simulink model "Part2_Solution"  (R2025a)
settings: Solver=VariableStepAuto  StopTime=5000
InitFcn:
  | addpath(fullfile(fileparts(get_param(bdroot,'FileName')),'..','..','AIEngine_Library','common','matlab')); CreateFilter;
undefined symbols (not defined in the file): Asymmetric, cfi, hb1, hb2, hb3, S, Shift1, Shift2, Shift3, ShiftCF, vsva2197, xcvc1902
libraries: aieDSP x4, aieBasic x3, dspmlti4 x3, aieUtilities x2, dspobslib x1, vmcUtilities x1
settings Model: Creator=robg  LastModifiedBy=robg
settings DebuggingCC: UnconnectedInputMsg=warning  UnconnectedOutputMsg=warning  UnconnectedLineMsg=warning
settings ModelReferenceCC: EnableRefExpFcnMdlSchedulingChecks=on
settings RTWCC: GPUComputeCapability=3.5  DLArmComputeVersion=19.05

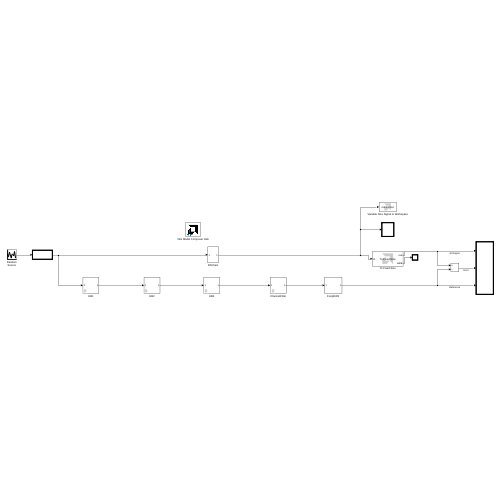
[thumbnail: Simulink's stored preview of the top-level diagram]
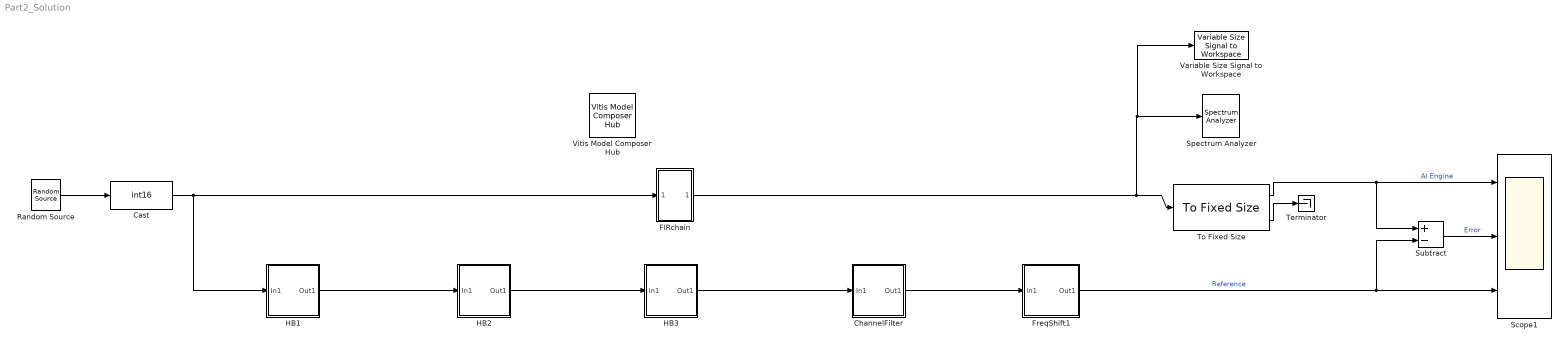
== system Part2_Solution ==
  Cast : DataTypeConversion  OutDataTypeStr=int16  SaturateOnIntegerOverflow=off  RndMeth=Floor
  ChannelFilter : Subsystem  mask{COEFFS=cfi, Shift=ShiftCF}
      mask prompts: COEFFS "Coefficients"; Shift "Final Shift"
  FIRchain : Subsystem
  FreqShift1 : Subsystem
  HB1 : Subsystem  mask{COEFFS=hb1, Shift=Shift1}
      mask prompts: COEFFS "Coefficients"; Shift "Final Shift"
  HB2 : Subsystem  mask{COEFFS=hb2, Shift=Shift2}
      mask prompts: COEFFS "Coefficients"; Shift "Final Shift"
  HB3 : Subsystem  mask{COEFFS=hb3, Shift=Shift3}
      mask prompts: COEFFS "Coefficients"; Shift "Final Shift"
  Random Source : dspobslib/Random Source  SrcType=Uniform  NormMethod=Ziggurat  CltLength=12  MinVal=-30000  MaxVal=30000  MeanVal=0  VarVal=1  RepMode=Not repeatable  rawSeed=1  IsInherit=off  SampMode=Discrete  SampTime=1  SampFrame=2048  DataType=Double  OutComplex=Complex  OutputFrames=off
  Scope1 : Scope  NumInputPorts=3
      settings: ActiveDisplayYMinimum=-22403.25  ActiveDisplayYMaximum=20249.25
  Spectrum Analyzer : SpectrumAnalyzer  WindowPosition=[236 135 808 450]  Visible=on  SampleRate=0.125  Span=0.125  StartFrequency=-0.0625  StopFrequency=0.0625  AveragingMethod=Exponential  YLimits=[32.3623,86.1256]  ChannelNames="[\"\"]"  AllowFFTLengthLessThanSamplesPerUpdate=on  DefaultConfigurationName=spbscopes.SpectrumAnalyzerBlockCfg
  Subtract : Sum  Inputs=+-
  Terminator : Terminator
  To Fixed Size : aieUtilities/To Fixed Size  Mode=Produce a valid output signal  OutputSize=256  CopyMethod=Buffer samples to form output  HasStatusOutput=on
  Variable Size Signal to Workspace : aieUtilities/Variable Size Signal to Workspace  VariableNameMask=simout
  Vitis Model Composer Hub : vmcUtilities/Vitis Model Composer Hub  Tag=genX  CodeGeneration=off  SubsystemName=FIRchain  StartColumn=1  NumberOfColumns=1  TargetDirectory=./code  exportDesign=off  analyzeDesign=off  validateDesignOnHw=off  ExportType=HW Code  IpVendor=xilinx.com  IpLibrary=hls  IpVersion=1.0  IpHWLanguage=Verilog  AieCompilerOptions={}  AieSimulatorOptions={}  CreateTestbench=off  TestbenchStackSize=10  RunRtlSim=off  RunCSim=off  RunAieSim=off  enableSimulationTimeout=on  enableGraphIterations=on  AieSimTimeout=50000  AieGraphIterations=-1  RunAieSimProfiling=off  LaunchVitisAnalyzer=off  PlotOutput=off  RunX86Sim=off  X86SimTimeout=10  GenHwImage=off  GenLibadfXo=off  GenHwValidationCode=off  PlatformType=Specify Platform  Platform=/proj/xbuilds/SWIP/2023.1_0417_2103/installs/lin64/Vitis/2023.1/base_platforms/xilinx_vck190_base_202310_1/xilinx_vck190_base_202310_1.xpfm  HwSystemType=Baremetal  HwValidationTarget=hw  ProjDevice=xcvc1902-vsva2197-2MP-e-S  ProjDevicePart=xcvc1902-vsva2197-2MP-e-S  AIEType=AIE  SamplePeriod=-1  ClockFrequency=200  DataPathParallelism=1  xilinxfamily=versalaicore  part=xcvc1902  speed=-2MP-e-S  package=vsva2197  directory=./netlist  testbench=off  incr_netlist=off  synthesis_tool=Vivado  clock_wrapper=Clock Enables  dbl_ovrd=According to Block Masks  dcm_input_clock_period=10  sysclk_period=10  simulink_period=1  eval_field=0  LogFileName=/proj/xcoswmktg/robg/git/AIEngine_Library/06-Hardware_Validation/work/code/model_composer.log  NThreads=4
  wires:
  Random Source/1 -> Cast/1
  Cast/1 -> FIRchain/1(In1), HB1/1(In1)
  To Fixed Size/2 -> Terminator/1
  Subtract/1 -> Scope1/2  "Error"
  To Fixed Size/1 -> Subtract/1, Scope1/1  "AI Engine"
  HB1/1(Out1) -> HB2/1(In1)
  HB2/1(Out1) -> HB3/1(In1)
  HB3/1(Out1) -> ChannelFilter/1(In1)
  ChannelFilter/1(Out1) -> FreqShift1/1(In1)
  FreqShift1/1(Out1) -> Subtract/2, Scope1/3  "Reference"
  FIRchain/1(Out1) -> Variable Size Signal to Workspace/1, Spectrum Analyzer/1, To Fixed Size/1

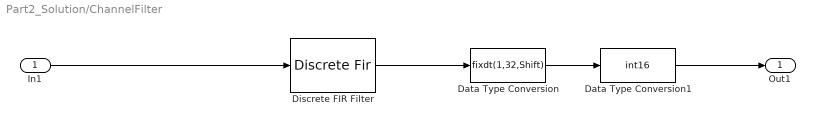
== system Part2_Solution/ChannelFilter ==
  In1 : Inport
  Data Type Conversion : DataTypeConversion  OutDataTypeStr=fixdt(1,32,Shift)  ConvertRealWorld=Stored Integer (SI)  SaturateOnIntegerOverflow=off  RndMeth=Floor
  Data Type Conversion1 : DataTypeConversion  OutDataTypeStr=int16  RndMeth=Floor
  Discrete FIR Filter : DiscreteFir  Coefficients=COEFFS  InputProcessing=Columns as channels (frame based)
  Out1 : Outport
  wires:
  Data Type Conversion/1 -> Data Type Conversion1/1
  In1/1 -> Discrete FIR Filter/1
  Discrete FIR Filter/1 -> Data Type Conversion/1
  Data Type Conversion1/1 -> Out1/1

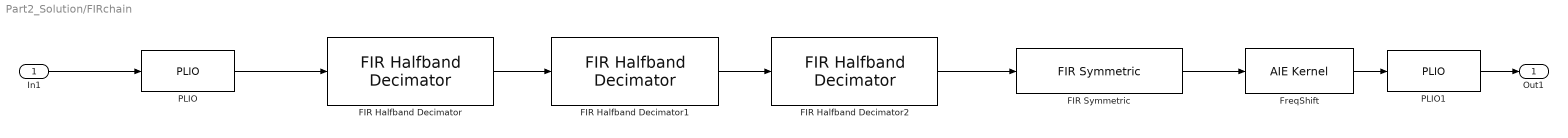
== system Part2_Solution/FIRchain ==
  In1 : Inport
  FIR Halfband Decimator : aieDSP/FIR Halfband Decimator  data_type=cint16  coef_type=int16  use_coeff_reload=off  dual_ip=off  num_outputs=off  coeff=hb1_aie  fir_length=31  input_window_size=2048  shift_val=Shift1  rnd_mode=Floor  sat_mode=1-Asymmetric  deci_poly=1  casc_length=2  AIE_VARIANT=1  TP_API=0  ssr=1  blockJsonConstraints=[]  blockJsonConstraintsInternal=[]  spec=vmc_fir_decimate_hb.json  SerializedMaskParamNames=[]  SerializedMaskParamValues=[]  SerializedMaskParamVisibilities=[]  block_type=FIR Halfband Decimator  SerializedMaskParamDataypes=typename|typename|uint|uint|uint|coef_type|uint|uint|uint|uint|uint|uint|uint|uint|uint|uint  SerializedMaskParamEnumStrArr=0|0|0|0|0|0|0|0|0|Floor,Ceiling,Round to positive infinity,Round to negative infinity,Round symmetrical to infinity,Round symmetrical to zero,Round convergent to even,Round convergent to odd|0-None,1-Asymmetric,3-Symmetric|0|0|0|0|0  SerializedMaskParamEnumValArr=0|0|0|0|0|0|0|0|0|0,1,2,3,4,5,6,7|0,1,3|0|0|0|0|0  SerializedMaskParamVectorArr=0|0|0|0|0|1|0|0|0|0|0|0|0|0|0|0  SerializedMaskParamKeys=TT_DATA|TT_COEFF|TP_USE_COEFF_RELOAD|TP_DUAL_IP|TP_NUM_OUTPUTS|coeff|TP_FIR_LEN|TP_INPUT_WINDOW_VSIZE|TP_SHIFT|TP_RND|TP_SAT|TP_PARA_DECI_POLY|TP_CASC_LEN|AIE_VARIANT|TP_API|TP_SSR
  FIR Halfband Decimator1 : aieDSP/FIR Halfband Decimator  data_type=cint16  coef_type=int16  use_coeff_reload=off  dual_ip=off  num_outputs=off  coeff=hb2_aie  fir_length=31  input_window_size=1024  shift_val=Shift2  rnd_mode=Floor  sat_mode=1-Asymmetric  deci_poly=1  casc_length=2  AIE_VARIANT=1  TP_API=0  ssr=1  blockJsonConstraints=[]  blockJsonConstraintsInternal=[]  spec=vmc_fir_decimate_hb.json  SerializedMaskParamNames=[]  SerializedMaskParamValues=[]  SerializedMaskParamVisibilities=[]  block_type=FIR Halfband Decimator  SerializedMaskParamDataypes=typename|typename|uint|uint|uint|coef_type|uint|uint|uint|uint|uint|uint|uint|uint|uint|uint  SerializedMaskParamEnumStrArr=0|0|0|0|0|0|0|0|0|Floor,Ceiling,Round to positive infinity,Round to negative infinity,Round symmetrical to infinity,Round symmetrical to zero,Round convergent to even,Round convergent to odd|0-None,1-Asymmetric,3-Symmetric|0|0|0|0|0  SerializedMaskParamEnumValArr=0|0|0|0|0|0|0|0|0|0,1,2,3,4,5,6,7|0,1,3|0|0|0|0|0  SerializedMaskParamVectorArr=0|0|0|0|0|1|0|0|0|0|0|0|0|0|0|0  SerializedMaskParamKeys=TT_DATA|TT_COEFF|TP_USE_COEFF_RELOAD|TP_DUAL_IP|TP_NUM_OUTPUTS|coeff|TP_FIR_LEN|TP_INPUT_WINDOW_VSIZE|TP_SHIFT|TP_RND|TP_SAT|TP_PARA_DECI_POLY|TP_CASC_LEN|AIE_VARIANT|TP_API|TP_SSR
  FIR Halfband Decimator2 : aieDSP/FIR Halfband Decimator  data_type=cint16  coef_type=int16  use_coeff_reload=off  dual_ip=off  num_outputs=off  coeff=hb3_aie  fir_length=31  input_window_size=512  shift_val=Shift3  rnd_mode=Floor  sat_mode=1-Asymmetric  deci_poly=1  casc_length=2  AIE_VARIANT=1  TP_API=0  ssr=1  blockJsonConstraints=[]  blockJsonConstraintsInternal=[]  spec=vmc_fir_decimate_hb.json  SerializedMaskParamNames=[]  SerializedMaskParamValues=[]  SerializedMaskParamVisibilities=[]  block_type=FIR Halfband Decimator  SerializedMaskParamDataypes=typename|typename|uint|uint|uint|coef_type|uint|uint|uint|uint|uint|uint|uint|uint|uint|uint  SerializedMaskParamEnumStrArr=0|0|0|0|0|0|0|0|0|Floor,Ceiling,Round to positive infinity,Round to negative infinity,Round symmetrical to infinity,Round symmetrical to zero,Round convergent to even,Round convergent to odd|0-None,1-Asymmetric,3-Symmetric|0|0|0|0|0  SerializedMaskParamEnumValArr=0|0|0|0|0|0|0|0|0|0,1,2,3,4,5,6,7|0,1,3|0|0|0|0|0  SerializedMaskParamVectorArr=0|0|0|0|0|1|0|0|0|0|0|0|0|0|0|0  SerializedMaskParamKeys=TT_DATA|TT_COEFF|TP_USE_COEFF_RELOAD|TP_DUAL_IP|TP_NUM_OUTPUTS|coeff|TP_FIR_LEN|TP_INPUT_WINDOW_VSIZE|TP_SHIFT|TP_RND|TP_SAT|TP_PARA_DECI_POLY|TP_CASC_LEN|AIE_VARIANT|TP_API|TP_SSR
  FIR Symmetric : aieDSP/FIR Symmetric  data_type=cint16  coef_type=int16  use_coeff_reload=off  dual_ip=off  num_outputs=off  coeff=cfi_aie  fir_length=length(cfi)  input_window_size=256  shift_val=ShiftCF  rnd_mode=Floor  sat_mode=1-Asymmetric  casc_length=3  AIE_VARIANT=1  TP_API=0  ssr=1  blockJsonConstraints=[]  blockJsonConstraintsInternal=[]  spec=vmc_fir_sr_sym.json  SerializedMaskParamNames=[]  SerializedMaskParamValues=[]  SerializedMaskParamVisibilities=[]  block_type=FIR Symmetric  SerializedMaskParamDataypes=typename|typename|uint|uint|uint|coef_type|uint|uint|uint|uint|uint|uint|uint|uint|uint  SerializedMaskParamEnumStrArr=0|0|0|0|0|0|0|0|0|Floor,Ceiling,Round to positive infinity,Round to negative infinity,Round symmetrical to infinity,Round symmetrical to zero,Round convergent to even,Round convergent to odd|0-None,1-Asymmetric,3-Symmetric|0|0|0|0  SerializedMaskParamEnumValArr=0|0|0|0|0|0|0|0|0|0,1,2,3,4,5,6,7|0,1,3|0|0|0|0  SerializedMaskParamVectorArr=0|0|0|0|0|1|0|0|0|0|0|0|0|0|0  SerializedMaskParamKeys=TT_DATA|TT_COEFF|TP_USE_COEFF_RELOAD|TP_DUAL_IP|TP_NUM_OUTPUTS|coeff|TP_FIR_LEN|TP_INPUT_WINDOW_VSIZE|TP_SHIFT|TP_RND|TP_SAT|TP_CASC_LEN|AIE_VARIANT|TP_API|TP_SSR
  FreqShift : aieBasic/AIE Kernel  KernelAllAttrs=|  PortNames={'in'; 'out'}  PortSerializedTypes={'{Q2{R{Tadf::input_buffer{1{t{Scint16}}}}}}'; '{Q2{R{Tadf::output_buffer{1{t{Scint16}}}}}}'}  PortWindowSizes={2.560000000000000000e+02, 2.560000000000000000e+02}  PortWindowMargins={0.000000000000000000e+00, 0.000000000000000000e+00}  PortSynchronicities={'sync', 'sync'}  PortSignalSizes={0.000000000000000000e+00; 0.000000000000000000e+00}  FunctionTemplateSpecKind=implicit  FunctionTemplateParamNames={'FRAME_LENGTH'}  FunctionTemplateParamKinds={'nontype'}  FunctionTemplateParamTypes={'int'}  FunctionTemplateParamValues={'256'}  FunctionIndex=1  FunctionTabVisible=on  FunctionTemplateParamsVisible=on  PreSSR=1  isImport=false  FunctionDeclTypeOptions=|  FunctionDecl=|  FunctionTemplateParams={ 'FRAME_LENGTH', 'int', '256' }  FunctionTemplateParamsEnables={'off', 'off', 'on'}  PortAttrs={ 'input', 'in', 'adf::input_buffer< cint16 > & restrict', '256', '0', 'sync', ''; 'output', 'out', 'adf::output_buffer< cint16 > & restrict', '256', '', 'sync', '' }  PortAttrsEnables={'off', 'off', 'off', 'on', 'off', 'off', 'off';'off', 'off', 'off', 'on', 'off', 'off', 'off'}  SampleTime=-1  KernelHeaderFile=FreqShift.h  KernelFunction=FreqShift  KernelSourceFile=FreqShift.cpp  KernelSearchPaths={}  PreProcOptions={}  ssr=1  blockJsonConstraints=[]
      KernelAllAttrs=|
      | s[12;12;9;9;19;14;21;23;21;23;24;21;15;17;12;24;26;26;26;27;28;9;21;23;23;23;24;25;14;19;19;29]@FunctionNameDeclFileNamePortNamesPortTypesPortSerializedTypesPortDirectionsPortWindowSizeEnablesPortWindowMarginEnablesPortBufferSizeEnablesPortBufferMarginEnablesPortSynchronicityEnablesPortSignalSizeEnablesPortBufferSizesPortBufferMarginsFunctionDeclFunctionTemplateSpecKindFunctionTemplateParamNamesFunctionTemplateParamKindsFunctionTemplateParamTypesFunctionTemplateParamValuesFunctionTemplateParamEnablesClassDeclClassTemplateSpecKindClassTemplateParamNamesClassTemplateParamKindsClassTemplateParamTypesClassTemplateParamValuesClassTemplateParamEnablesClassCtorDeclsClassCtorParamNamesClassCtorParamTypesClassCtorParamSerializedTypes[1 1]@C[32 1]@t9@FreqShiftt17@../../FreqShift.hC[2 1]@t2@int3@outC[2 1]@t38@adf::input_buffer< cint16 > & restrictt39@adf::output_buffer< cint16 > & restrictC[2 1]@t42@{Q2{R{Tadf::input_buffer{1{t{Scint16}}}}}}t43@{Q2{R{Tadf::output_buffer{1{t{Scint16}}}}}}C[2 1]@t5@inputt6@outputC[2 1]@l1@l1@C[2 1]@l1@l0@C[2 1]@l1@l1@C[2 1]@l0@l0@C[2 1]@l1@l1@C[2 1]@l0@l0@C[2 1]@nnC[2 1]@nnt133@template < int FRAME_LENGTH > 
      | void FreqShift(adf::input_buffer< cint16 > & restrict in, adf::output_buffer< cint16 > & restrict out)t8@implicitC[1 1]@t12@FRAME_LENGTHC[1 1]@t7@nontypeC[1 1]@t3@intC[1 1]@nC[1 1]@l1@nne[0 1]@e[0 1]@e[0 1]@e[0 1]@e[0 1]@e[0 1]@e[0 1]@e[0 1]@e[0 1]@
      FunctionDeclTypeOptions=|
      | C[1 1]@t135@template < int FRAME_LENGTH > 
      | void FreqShift(adf::input_buffer< cint16 > && restrict in, adf::output_buffer< cint16 > && restrict out)
      FunctionDecl=|
      | template < int FRAME_LENGTH > 
      | void FreqShift(adf::input_buffer< cint16 > && restrict in, adf::output_buffer< cint16 > && restrict out)
  PLIO : aieBasic/PLIO  PlioWidth=128  PlioFreqSpec=on  PlioFreq=500  ColLocation=0  channel=0  blockJsonConstraints=[]  deprecateConstraints=0
  PLIO1 : aieBasic/PLIO  PlioWidth=128  PlioFreqSpec=on  PlioFreq=500  ColLocation=0  channel=0  blockJsonConstraints=[]  deprecateConstraints=0
  Out1 : Outport
  wires:
  In1/1 -> PLIO/1
  FIR Halfband Decimator1/1 -> FIR Halfband Decimator2/1
  FreqShift/1 -> PLIO1/1
  FIR Symmetric/1 -> FreqShift/1
  FIR Halfband Decimator2/1 -> FIR Symmetric/1
  FIR Halfband Decimator/1 -> FIR Halfband Decimator1/1
  PLIO/1 -> FIR Halfband Decimator/1
  PLIO1/1 -> Out1/1

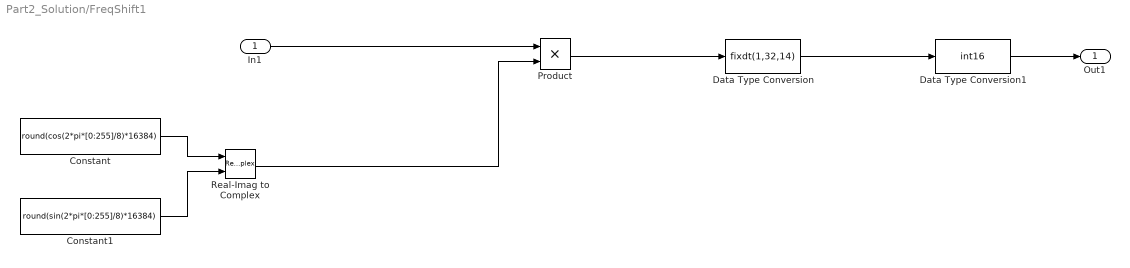
== system Part2_Solution/FreqShift1 ==
  In1 : Inport
  Constant : Constant  Value=round(cos(2*pi*[0:255]/8)*16384)  SampleTime=2048
  Constant1 : Constant  Value=round(sin(2*pi*[0:255]/8)*16384)  SampleTime=2048
  Data Type Conversion : DataTypeConversion  OutDataTypeStr=fixdt(1,32,14)  ConvertRealWorld=Stored Integer (SI)  SaturateOnIntegerOverflow=off  RndMeth=Floor
  Data Type Conversion1 : DataTypeConversion  OutDataTypeStr=int16  RndMeth=Floor
  Product : Product
  Real-Imag to Complex : RealImagToComplex
  Out1 : Outport
  wires:
  In1/1 -> Product/1
  Product/1 -> Data Type Conversion/1
  Real-Imag to Complex/1 -> Product/2
  Data Type Conversion1/1 -> Out1/1
  Constant/1 -> Real-Imag to Complex/1
  Constant1/1 -> Real-Imag to Complex/2
  Data Type Conversion/1 -> Data Type Conversion1/1

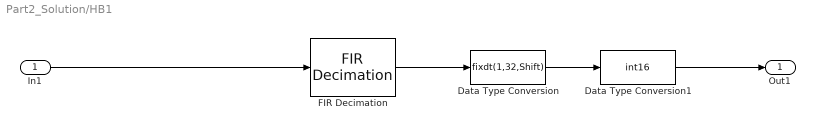
== system Part2_Solution/HB1 ==
  In1 : Inport
  Data Type Conversion : DataTypeConversion  OutDataTypeStr=fixdt(1,32,Shift)  ConvertRealWorld=Stored Integer (SI)  SaturateOnIntegerOverflow=off  RndMeth=Floor
  Data Type Conversion1 : DataTypeConversion  OutDataTypeStr=int16  RndMeth=Floor
  FIR Decimation : dspmlti4/FIR Decimation  FilterSource=Dialog parameters  h=COEFFS  D=2  filtStruct=Direct form  FilterObject=FDECIM  InputProcessing=Columns as channels (frame based)  framing=Enforce single-rate processing  AllowArbitraryInputLength=off  inputOffset=0  outputBufInitCond=0  roundingMode=Floor  overflowMode=off  firstCoeffDataTypeStr=Inherit: Same word length as input  firstCoeffMin=[]  firstCoeffMax=[]  firstCoeffLastDataTypeStr=Inherit: Same word length as input  outputDataTypeStr=Inherit: Same as accumulator  outputMin=[]  outputMax=[]  outputLastDataTypeStr=Inherit: Same as accumulator
  Out1 : Outport
  wires:
  Data Type Conversion/1 -> Data Type Conversion1/1
  In1/1 -> FIR Decimation/1
  FIR Decimation/1 -> Data Type Conversion/1
  Data Type Conversion1/1 -> Out1/1

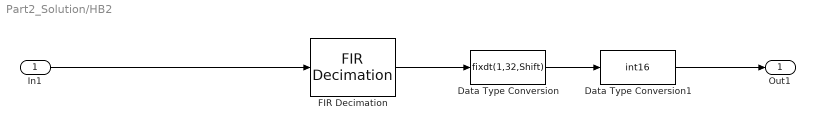
== system Part2_Solution/HB2 ==
  In1 : Inport
  Data Type Conversion : DataTypeConversion  OutDataTypeStr=fixdt(1,32,Shift)  ConvertRealWorld=Stored Integer (SI)  SaturateOnIntegerOverflow=off  RndMeth=Floor
  Data Type Conversion1 : DataTypeConversion  OutDataTypeStr=int16  RndMeth=Floor
  FIR Decimation : dspmlti4/FIR Decimation  FilterSource=Dialog parameters  h=COEFFS  D=2  filtStruct=Direct form  FilterObject=FDECIM  InputProcessing=Columns as channels (frame based)  framing=Enforce single-rate processing  AllowArbitraryInputLength=off  inputOffset=0  outputBufInitCond=0  roundingMode=Floor  overflowMode=off  firstCoeffDataTypeStr=Inherit: Same word length as input  firstCoeffMin=[]  firstCoeffMax=[]  firstCoeffLastDataTypeStr=Inherit: Same word length as input  outputDataTypeStr=Inherit: Same as accumulator  outputMin=[]  outputMax=[]  outputLastDataTypeStr=Inherit: Same as accumulator
  Out1 : Outport
  wires:
  Data Type Conversion/1 -> Data Type Conversion1/1
  In1/1 -> FIR Decimation/1
  FIR Decimation/1 -> Data Type Conversion/1
  Data Type Conversion1/1 -> Out1/1

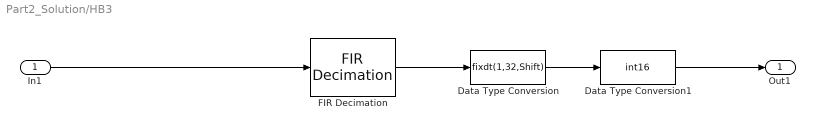
== system Part2_Solution/HB3 ==
  In1 : Inport
  Data Type Conversion : DataTypeConversion  OutDataTypeStr=fixdt(1,32,Shift)  ConvertRealWorld=Stored Integer (SI)  SaturateOnIntegerOverflow=off  RndMeth=Floor
  Data Type Conversion1 : DataTypeConversion  OutDataTypeStr=int16  RndMeth=Floor
  FIR Decimation : dspmlti4/FIR Decimation  FilterSource=Dialog parameters  h=COEFFS  D=2  filtStruct=Direct form  FilterObject=FDECIM  InputProcessing=Columns as channels (frame based)  framing=Enforce single-rate processing  AllowArbitraryInputLength=off  inputOffset=0  outputBufInitCond=0  roundingMode=Floor  overflowMode=off  firstCoeffDataTypeStr=Inherit: Same word length as input  firstCoeffMin=[]  firstCoeffMax=[]  firstCoeffLastDataTypeStr=Inherit: Same word length as input  outputDataTypeStr=Inherit: Same as accumulator  outputMin=[]  outputMax=[]  outputLastDataTypeStr=Inherit: Same as accumulator
  Out1 : Outport
  wires:
  Data Type Conversion1/1 -> Out1/1
  FIR Decimation/1 -> Data Type Conversion/1
  In1/1 -> FIR Decimation/1
  Data Type Conversion/1 -> Data Type Conversion1/1
